simulink model "MinSeg_Controller_v2"  (R2014b)
settings: Solver=FixedStepDiscrete  SolverMode=SingleTasking  StartTime=0.0  StopTime=inf  FixedStep=TS  RelTol=1e-3
values from neighbouring files (symbols this model uses):
  ES = -C2DEG*D2R    (= -0.00872664625997)    [MinSeg_Parameters.m]    (also in MinSeg_Parameters_v2.m; MinSeg_Parameters_v3.m)
  GS = GyroS*D2R    (= 0.000155832968928)    [MinSeg_Parameters.m]    (also in MinSeg_Parameters_v2.m; MinSeg_Parameters_v3.m)
  Ki = 1*[-r_w -r_w*0 1 1*0]    [MinSeg_Parameters.m]    (also in MinSeg_Parameters_v2.m; MinSeg_Parameters_v3.m)
  KLQRC = KLQR.*[-r_w -r_w 1 1]    [MinSeg_Parameters.m]    (also in MinSeg_Parameters_v2.m; MinSeg_Parameters_v3.m)
  TS = .03    (= 0.03)    [MinSeg_Parameters.m]    (also in MinSeg_Parameters_v2.m; MinSeg_Parameters_v3.m = 0.005)
  tstart = 2    [MinSeg_Parameters.m]    (also in MinSeg_Parameters_v2.m; MinSeg_Parameters_v3.m)
  V2DCB = 1/DCB2V    (= 42.5)    [MinSeg_Parameters.m]    (also in MinSeg_Parameters_v2.m = 28.3333333333; MinSeg_Parameters_v3.m = 28.3333333333)
libraries: arduinolib x3, simulink x2
settings Model: FPTRunName=FPA_Reference  SimulationMode=external  ExtModeTrigDuration=2  Creator=Alec  LastModifiedBy=lq561d
settings OptimizationCC: ExpressionDepthLimit=2147483647  OptimizeModelRefInitCode=on  LifeSpan=1
settings DebuggingCC: UnderspecifiedInitializationDetection=Classic  MergeDetectMultiDrivingBlocksExec=none  SolverPrmCheckMsg=none  StateNameClashWarn=warning
settings HardwareCC: ProdBitPerInt=16  ProdBitPerPointer=8  ProdIntDivRoundTo=Zero  ProdEndianess=LittleEndian  ProdWordSize=8  ProdHWDeviceType=Atmel->AVR
settings RTWCC: SystemTargetFile=realtime.tlc  GenerateMakefile=off  TemplateMakefile=realtime.tmf  Description=Real-Time Toolbox  RTWVerbose=off  ProcessScript=realtime_make_rtw_hook
settings CodeAppCC: CustomSymbolStrType=$N$R$M  InternalIdentifier=Classic
settings STFCustomTargetCC: TargetLibSuffix=.a  GenerateSampleERTMain=on  ERTCustomFileBanners=on  SupportNonInlinedSFcns=off  SupportVariableSizeSignals=on  MATLABClassNameForMDSCustomization=Simulink.SoftwareTarget.ERTCustomization  GRTInterface=off  SystemTargetFile=realtime.tlc
settings ERTTargetCC: GenerateSampleERTMain=on  ParMdlRefBuildCompliant=off  CompOptLevelCompliant=off  ConcurrentExecutionCompliant=off  CombineOutputUpdateFcns=off  ERTFirstTimeCompliant=off  SupportContinuousTime=on  SupportVariableSizeSignals=on  ModelStepFunctionPrototypeControlCompliant=off  CPPClassGenCompliant=off  ExtModeTransport=3  ExtModeMexFile=ext_serial_win32_comm  ExtModeMexArgs=0 7 115200  InlinedParameterPlacement=NonHierarchical  ERTSrcFileBannerTemplate=realtime_code_template.cgt  ERTHdrFileBannerTemplate=realtime_code_template.cgt  ERTDataSrcFileTemplate=realtime_code_template.cgt  ERTDataHdrFileTemplate=realtime_code_template.cgt  ERTCustomFileTemplate=realtime_file_process.tlc

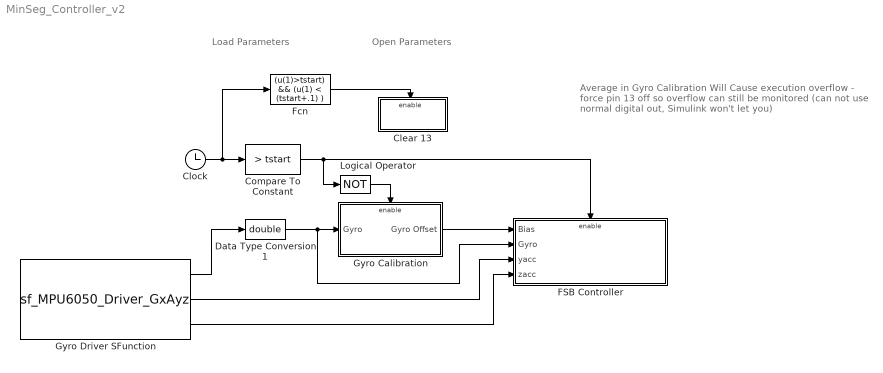
== system MinSeg_Controller_v2 ==
  note: Average in Gyro Calibration Will
      | Cause execution overflow - force pin 13 off
      | so overflow can still be monitored (can not use normal
      | digital out, Simulink won't let you)
  note: Load Parameters
  note: Open Parameters
  "Clear 13 " : Subsystem  TreatAsAtomicUnit=on
  Clock : Clock
  Compare To Constant : simulink/Logic and Bit Operations/Compare To Constant  relop=>  const=tstart  OutDataTypeStr=boolean
  Data Type Conversion1 : DataTypeConversion  OutDataTypeStr=double
  FSB Controller : Subsystem
  Fcn : Fcn  Expr=(u(1)>tstart) && (u(1) < (tstart+.1) )
  Gyro Calibration : Subsystem  TreatAsAtomicUnit=on
  Gyro Driver SFunction : S-Function  InitFcn=try, set_param(gcb,'FunctionName','sf_MPU6050_Driver_GxAyz'), end  FunctionName=sf_MPU6050_Driver_GxAyz  SFunctionModules=sf_MPU6050_Driver_GxAyz_wrapper  EnableBusSupport=off  mask(S-Function Builder){}
      mask help: Simulink:masks:SFunctionBuilder_MD
      mask init:
      | val = [[.9  0.75 0.75 1 1 .9 .9 1]',[1 1 0.75 0.75 .9 .9 1 .9]'];try , sys = get_param(gcb,'SfunBuilderFcnName');if isempty(sys), sys = get_param(gcb,'FunctionName'); end,catch, sys = get_param(gcb,'FunctionName'); end
      settings: CopyFcn=set_param(gcbh,'LinkStatus','none')  PreSaveFcn=try, set_param(gcb,'FunctionName','sf_MPU6050_Driver_GxAyz'), end  OpenFcn=sfunctionwizard(gcbh)
      mask Display: plot(val(:,1),val(:,2)),disp(sys), port_label('output',1,'x_vel'), port_label('output',2,'y_acc'), port_label('output',3,'z_acc')
  Logical Operator : Logic  Operator=NOT  AllPortsSameDT=off  OutDataTypeStr=boolean
  wires:
  Clock/1 -> Fcn/1, Compare To Constant/1
  Compare To Constant/1 -> Logical Operator/1, FSB Controller/Enable
  Gyro Calibration/1(Gyro Offset) -> FSB Controller/1(Bias)
  Gyro Driver SFunction/1 -> Data Type Conversion1/1
  Logical Operator/1 -> Gyro Calibration/Enable
  Data Type Conversion1/1 -> FSB Controller/2(Gyro), Gyro Calibration/1(Gyro)
  Fcn/1 -> "Clear 13 "/Enable
  Gyro Driver SFunction/2 -> FSB Controller/3("yacc ")
  Gyro Driver SFunction/3 -> FSB Controller/4("zacc ")

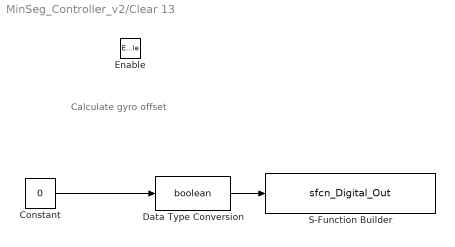
== system MinSeg_Controller_v2/Clear 13  ==
  note: Calculate gyro offset
  Enable : EnablePort
  Constant : Constant  Value=0
  Data Type Conversion : DataTypeConversion  OutDataTypeStr=boolean
  S-Function Builder : S-Function  InitFcn=try, set_param(gcb,'FunctionName','sfcn_Digital_Out'), end  FunctionName=sfcn_Digital_Out  Parameters=uint8(13)  SFunctionModules=sfcn_Digital_Out_wrapper  EnableBusSupport=off  mask(S-Function Builder){}
      mask init: same as MinSeg_Controller_v2/Gyro Driver SFunction
      settings: CopyFcn=set_param(gcbh,'LinkStatus','none')  PreSaveFcn=try, set_param(gcb,'FunctionName','sfcn_Digital_Out'), end  OpenFcn=sfunctionwizard(gcbh)
      mask Display: plot(val(:,1),val(:,2)),disp(sys), port_label('input',1,'in')
  wires:
  Data Type Conversion/1 -> S-Function Builder/1
  Constant/1 -> Data Type Conversion/1

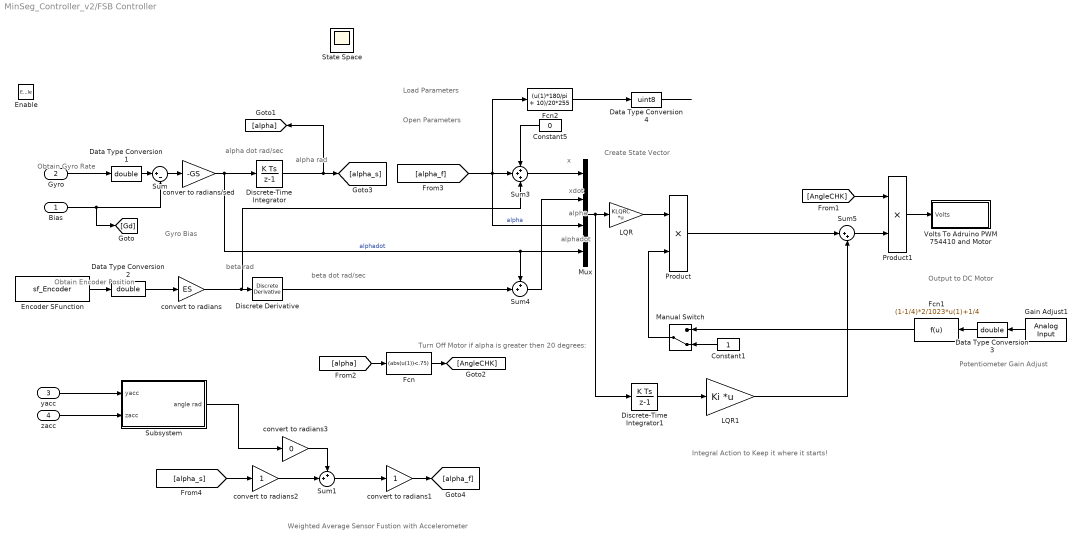
== system MinSeg_Controller_v2/FSB Controller ==
  note: Integral Action to Keep it where it starts!
  note: Weighted Average Sensor Fustion with Accelerometer
  note: Gyro
      | Bias
  note: Turn Off Motor if alpha is greater then 20 degrees:
  note: Output to DC Motor
  note: Create State Vector
  note: Obtain Encoder Position
  note: Obtain Gyro Rate
  note: xdot
  note: x
  note: beta
      | rad
  note: alpha dot
      | rad/sec
  note: alpha
      | rad
  note: beta dot
      | rad/sec
  note: alpha
  note: alphadot
  note: Load Parameters
  note: Open Parameters
  note: Potentiometer Gain Adjust
  Bias : Inport
  Gyro : Inport  Port=2
  "yacc " : Inport  Port=3
  "zacc " : Inport  Port=4
  Enable : EnablePort
  Constant1 : Constant
  Constant5 : Constant  Value=0
  Data Type Conversion1 : DataTypeConversion  OutDataTypeStr=double
  Data Type Conversion2 : DataTypeConversion  OutDataTypeStr=double
  Data Type Conversion3 : DataTypeConversion  OutDataTypeStr=double
  Data Type Conversion4 : DataTypeConversion  OutDataTypeStr=uint8
  Discrete Derivative : simulink/Discrete/Discrete Derivative  gainval=1.0  ICPrevScaledInput=0.0  InputProcessing=Inherited  OutMin=[]  OutMax=[]  OutDataType=fixdt(1, 16)  OutScaling=2^-10  DoSatur=off
  Discrete-Time Integrator : DiscreteIntegrator  SampleTime=TS
  Discrete-Time Integrator1 : DiscreteIntegrator  SampleTime=TS
  Encoder SFunction : S-Function  InitFcn=try, set_param(gcb,'FunctionName','sf_Encoder'), end  FunctionName=sf_Encoder  Parameters=uint8(0),uint8(18),uint8(19)  SFunctionModules=sf_Encoder_wrapper  EnableBusSupport=off  mask(S-Function Builder){}
      mask init: same as MinSeg_Controller_v2/Gyro Driver SFunction
      settings: CopyFcn=set_param(gcbh,'LinkStatus','none')  PreSaveFcn=try, set_param(gcb,'FunctionName','sf_Encoder'), end  OpenFcn=sfunctionwizard(gcbh)
      mask Display: plot(val(:,1),val(:,2)),disp(sys), port_label('output',1,'pos')
  Fcn : Fcn  Expr=(abs(u(1))<.75)
  Fcn1 : Fcn  Expr=(1-1/4)*2/1023*u(1)+1/4
  Fcn2 : Fcn  Expr="(u(1)*180/pi   + 10)/20*255"
  Gain Adjust1 : arduinolib/Analog Input  pinNumber=0  sampleTime=-1  blockPlatform=arduino
  LQR : Gain  Gain=KLQRC  Multiplication=Matrix(K*u)
  LQR1 : Gain  Gain=Ki  Multiplication=Matrix(K*u)
  Manual Switch : ManualSwitch  CurrentSetting=0
  Mux : Mux
  Product : Product  RndMeth=Zero
  Product1 : Product  RndMeth=Zero
  State Space : Scope  NumInputPorts=4
      settings: Floating=on  YMin=-7.5~-40~-0.45~-1.5  YMax=-5.5~20~-0.05~1.5  SaveName=ScopeData3
  Subsystem : Subsystem
  Sum : Sum  Inputs=|+-
  Sum1 : Sum  Inputs=++|
  Sum3 : Sum  Inputs=+++
  Sum4 : Sum  Inputs=++|
  Sum5 : Sum  Inputs=|++
  Volts To Adruino PWM 754410 and Motor : Subsystem
  conver to radians/sed : Gain  Gain=-GS
  convert to radians : Gain  Gain=ES  OutDataTypeStr=double
  convert to radians1 : Gain  OutDataTypeStr=double
  convert to radians2 : Gain  OutDataTypeStr=double
  convert to radians3 : Gain  Gain=0  OutDataTypeStr=double
  wires:
  Data Type Conversion3/1 -> Fcn1/1
  Gain Adjust1/1 -> Data Type Conversion3/1
  Sum3/1 -> Mux/1
  Data Type Conversion2/1 -> convert to radians/1
  Bias/1 -> [Gd], Sum/2
  Sum/1 -> conver to radians/sed/1
  Fcn/1 -> [AngleCHK]
  Encoder SFunction/1 -> Data Type Conversion2/1
  Mux/1 -> Discrete-Time Integrator1/1, LQR/1
  convert to radians/1 -> Discrete Derivative/1, Sum3/3
  Data Type Conversion1/1 -> Sum/1
  Gyro/1 -> Data Type Conversion1/1
  [alpha] -> Fcn/1
  Discrete Derivative/1 -> Sum4/2
  conver to radians/sed/1 -> Discrete-Time Integrator/1, Sum4/1, Mux/4  "alphadot"
  Sum4/1 -> Mux/2
  Discrete-Time Integrator/1 -> [alpha_s], [alpha]
  Constant5/1 -> Sum3/1
  Fcn2/1 -> Data Type Conversion4/1
  Data Type Conversion4/1 -> ?
  "yacc "/1 -> Subsystem/1(yacc)
  "zacc "/1 -> Subsystem/2(zacc)
  Subsystem/1(angle rad) -> convert to radians3/1
  [alpha_f] -> Mux/3, Fcn2/1, Sum3/2  "alpha"
  [alpha_s] -> convert to radians2/1
  Sum1/1 -> convert to radians1/1
  convert to radians1/1 -> [alpha_f]
  convert to radians2/1 -> Sum1/2
  convert to radians3/1 -> Sum1/1
  Discrete-Time Integrator1/1 -> LQR1/1
  Product/1 -> Sum5/1
  LQR/1 -> Product/1
  Sum5/1 -> Product1/2
  Product1/1 -> Volts To Adruino PWM 754410 and Motor/1(Volts)
  [AngleCHK] -> Product1/1
  LQR1/1 -> Sum5/2
  Manual Switch/1 -> Product/2
  Fcn1/1 -> Manual Switch/1
  Constant1/1 -> Manual Switch/2

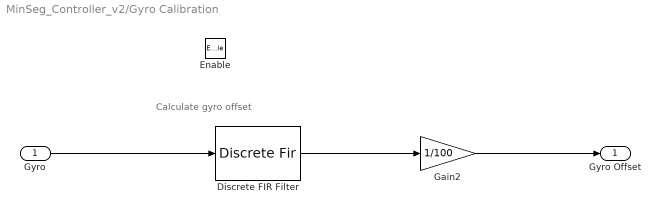
== system MinSeg_Controller_v2/Gyro Calibration ==
  note: Calculate gyro offset
  Gyro : Inport
  Enable : EnablePort
  Discrete FIR Filter : DiscreteFir  Coefficients=ones(1,100)
  Gain2 : Gain  Gain=1/100  OutDataTypeStr=Inherit: Same as input  ParamDataTypeStr=Inherit: Same as input
  Gyro Offset : Outport
  wires:
  Gyro/1 -> Discrete FIR Filter/1
  Discrete FIR Filter/1 -> Gain2/1
  Gain2/1 -> Gyro Offset/1

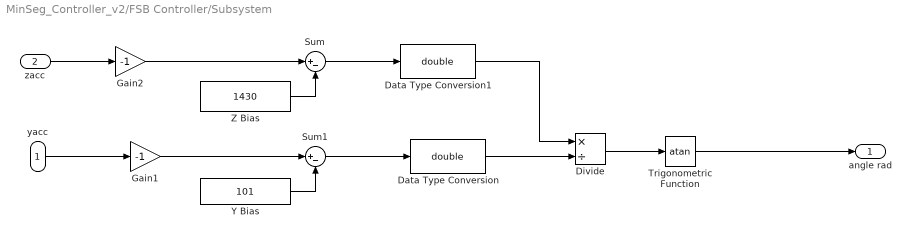
== system MinSeg_Controller_v2/FSB Controller/Subsystem ==
  yacc : Inport
  zacc : Inport  Port=2
  Data Type Conversion : DataTypeConversion  OutDataTypeStr=double
  Data Type Conversion1 : DataTypeConversion  OutDataTypeStr=double
  Divide : Product  Inputs=*/
  Gain1 : Gain  Gain=-1
  Gain2 : Gain  Gain=-1
  Sum : Sum  Inputs=|+-
  Sum1 : Sum  Inputs=|+-
  Trigonometric Function : Trigonometry  Operator=atan
  Y Bias : Constant  Value=101
  Z Bias : Constant  Value=1430
  angle rad : Outport
  wires:
  Sum1/1 -> Data Type Conversion/1
  Gain2/1 -> Sum/1
  Sum/1 -> Data Type Conversion1/1
  Z Bias/1 -> Sum/2
  Gain1/1 -> Sum1/1
  Y Bias/1 -> Sum1/2
  Trigonometric Function/1 -> angle rad/1
  Divide/1 -> Trigonometric Function/1
  zacc/1 -> Gain2/1
  yacc/1 -> Gain1/1
  Data Type Conversion1/1 -> Divide/1
  Data Type Conversion/1 -> Divide/2

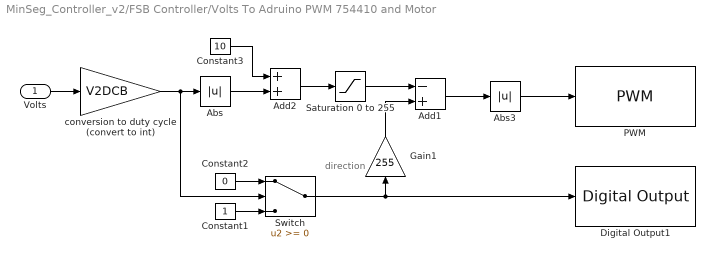
== system MinSeg_Controller_v2/FSB Controller/Volts To Adruino PWM 754410 and Motor ==
  note: direction
  Volts : Inport
  Abs : Abs
  Abs3 : Abs
  Add1 : Sum  Inputs=-+
  Add2 : Sum
  Constant1 : Constant
  Constant2 : Constant  Value=0
  Constant3 : Constant  Value=10
  Digital Output1 : arduinolib/Digital Output  pinNumber=6  blockPlatform=arduino
  Gain1 : Gain  Gain=255
  PWM : arduinolib/PWM  pinNumber=8  blockPlatform=arduino
  Saturation 0 to 255 : Saturate  UpperLimit=255  LowerLimit=0
  Switch : Switch
  conversion to duty cycle (convert to int) : Gain  Gain=V2DCB  OutDataTypeStr=int16
  wires:
  Volts/1 -> conversion to duty cycle (convert to int)/1
  Switch/1 -> Digital Output1/1, Gain1/1
  Constant2/1 -> Switch/1
  Constant1/1 -> Switch/3
  Gain1/1 -> Add1/2
  Add1/1 -> Abs3/1
  conversion to duty cycle (convert to int)/1 -> Switch/2, Abs/1
  Saturation 0 to 255/1 -> Add1/1
  Abs3/1 -> PWM/1
  Constant3/1 -> Add2/1
  Abs/1 -> Add2/2
  Add2/1 -> Saturation 0 to 255/1
